simulink model "NestedSubsystemModel_mdl"  (R2023b)
settings: Solver=VariableStepAuto  StartTime=0.0  StopTime=10.0  RelTol=1e-3
settings Model: Creator=jfrey  LastModifiedBy=jfrey

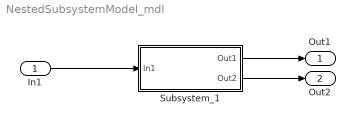
== system NestedSubsystemModel_mdl ==
  In1 : Inport
  Subsystem_1 : Subsystem
  Out1 : Outport
  Out2 : Outport  Port=2
  wires:
  In1/1 -> Subsystem_1/1(In1)
  Subsystem_1/1(Out1) -> Out1/1
  Subsystem_1/2(Out2) -> Out2/1

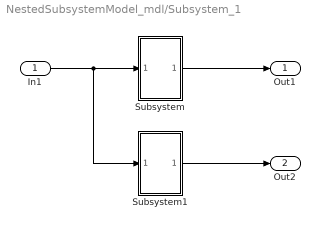
== system NestedSubsystemModel_mdl/Subsystem_1 ==
  In1 : Inport
  Subsystem : Subsystem
  Subsystem1 : Subsystem
  Out1 : Outport
  Out2 : Outport  Port=2
  wires:
  In1/1 -> Subsystem1/1(In1), Subsystem/1(In1)
  Subsystem/1(Out1) -> Out1/1
  Subsystem1/1(Out1) -> Out2/1

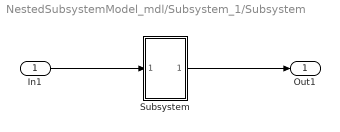
== system NestedSubsystemModel_mdl/Subsystem_1/Subsystem ==
  In1 : Inport
  Subsystem : Subsystem
  Out1 : Outport
  wires:
  In1/1 -> Subsystem/1(In1)
  Subsystem/1(Out1) -> Out1/1

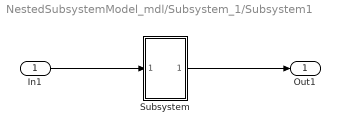
== system NestedSubsystemModel_mdl/Subsystem_1/Subsystem1 ==
  In1 : Inport
  Subsystem : Subsystem
  Out1 : Outport
  wires:
  In1/1 -> Subsystem/1(In1)
  Subsystem/1(Out1) -> Out1/1

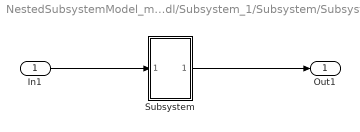
== system NestedSubsystemModel_mdl/Subsystem_1/Subsystem/Subsystem ==
  In1 : Inport
  Subsystem : Subsystem
  Out1 : Outport
  wires:
  In1/1 -> Subsystem/1(In1)
  Subsystem/1(Out1) -> Out1/1

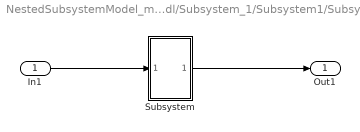
== system NestedSubsystemModel_mdl/Subsystem_1/Subsystem1/Subsystem ==
  In1 : Inport
  Subsystem : Subsystem
  Out1 : Outport
  wires:
  In1/1 -> Subsystem/1(In1)
  Subsystem/1(Out1) -> Out1/1

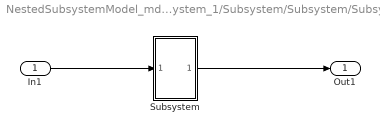
== system NestedSubsystemModel_mdl/Subsystem_1/Subsystem/Subsystem/Subsystem ==
  In1 : Inport
  Subsystem : Subsystem
  Out1 : Outport
  wires:
  In1/1 -> Subsystem/1(In1)
  Subsystem/1(Out1) -> Out1/1

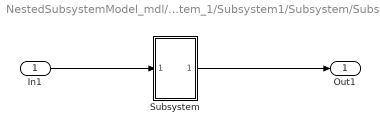
== system NestedSubsystemModel_mdl/Subsystem_1/Subsystem1/Subsystem/Subsystem ==
  In1 : Inport
  Subsystem : Subsystem
  Out1 : Outport
  wires:
  In1/1 -> Subsystem/1(In1)
  Subsystem/1(Out1) -> Out1/1

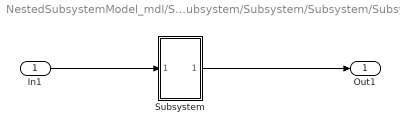
== system NestedSubsystemModel_mdl/Subsystem_1/Subsystem/Subsystem/Subsystem/Subsystem ==
  In1 : Inport
  Subsystem : Subsystem
  Out1 : Outport
  wires:
  In1/1 -> Subsystem/1(In1)
  Subsystem/1(Out1) -> Out1/1

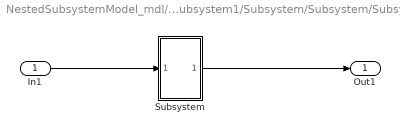
== system NestedSubsystemModel_mdl/Subsystem_1/Subsystem1/Subsystem/Subsystem/Subsystem ==
  In1 : Inport
  Subsystem : Subsystem
  Out1 : Outport
  wires:
  In1/1 -> Subsystem/1(In1)
  Subsystem/1(Out1) -> Out1/1

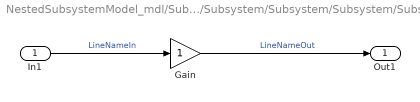
== system NestedSubsystemModel_mdl/Subsystem_1/Subsystem/Subsystem/Subsystem/Subsystem/Subsystem ==
  In1 : Inport
  Gain : Gain
  Out1 : Outport
  wires:
  In1/1 -> Gain/1  "LineNameIn"
  Gain/1 -> Out1/1  "LineNameOut"

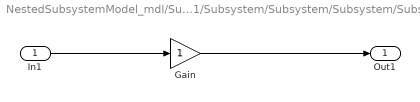
== system NestedSubsystemModel_mdl/Subsystem_1/Subsystem1/Subsystem/Subsystem/Subsystem/Subsystem ==
  In1 : Inport
  Gain : Gain
  Out1 : Outport
  wires:
  In1/1 -> Gain/1
  Gain/1 -> Out1/1
